simulink model "PIDcontroller"  (Simulink 6.5)
settings: Solver=FixedStepDiscrete  StartTime=0.0  StopTime=10.0  FixedStep=0.1  RelTol=1e-3
settings Model: Creator=AugustineBui  LastModifiedBy=AugustineBui
settings OptimizationCC: InitFltsAndDblsToZero=off
settings DebuggingCC: SignalResolutionControl=UseLocalSettings  StrictBusMsg=ErrorLevel1
settings HardwareCC: TargetHWDeviceType=32-bit Generic
settings GRTTargetCC: ExtModeInterfaceLevel=Level1

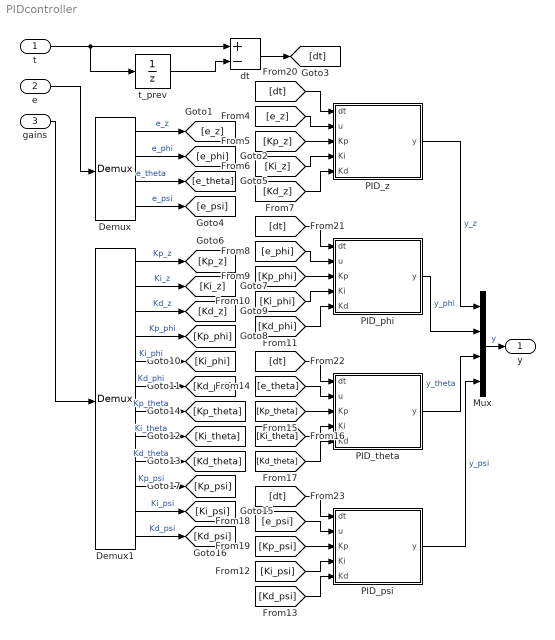
== system PIDcontroller ==
  t : Inport  PortDimensions=1  DataType=double
  e : Inport  Port=2  PortDimensions=4  DataType=double
  gains : Inport  Port=3  PortDimensions=12  DataType=double
  Demux : Demux
  Demux1 : Demux  Outputs=12
  Mux : Mux
  PID_phi : Subsystem
  PID_psi : Subsystem
  PID_theta : Subsystem
  PID_z : Subsystem
  dt : Sum  Inputs=+-
  t_prev : UnitDelay  X0=-0.5  SampleTime=-1
  y : Outport
  wires:
  [Kd_psi] -> PID_psi/5(Kd)
  [Ki_psi] -> PID_psi/4(Ki)
  [dt] -> PID_psi/1(dt)
  [e_psi] -> PID_psi/2(u)
  [Kp_psi] -> PID_psi/3(Kp)
  PID_psi/1(y) -> Mux/4  "y_psi"
  PID_theta/1(y) -> Mux/3  "y_theta"
  [Kd_theta] -> PID_theta/5(Kd)
  [Ki_theta] -> PID_theta/4(Ki)
  [dt] -> PID_theta/1(dt)
  [e_theta] -> PID_theta/2(u)
  [Kp_theta] -> PID_theta/3(Kp)
  PID_phi/1(y) -> Mux/2  "y_phi"
  [Kp_phi] -> PID_phi/3(Kp)
  [dt] -> PID_phi/1(dt)
  [dt] -> PID_z/1(dt)
  dt/1 -> [dt]
  [e_phi] -> PID_phi/2(u)
  t/1 -> t_prev/1, dt/1
  t_prev/1 -> dt/2
  e/1 -> Demux/1
  gains/1 -> Demux1/1
  Demux/1 -> [e_z]  "e_z"
  Demux/2 -> [e_phi]  "e_phi"
  Demux/3 -> [e_theta]  "e_theta"
  Demux/4 -> [e_psi]  "e_psi"
  Demux1/1 -> [Kp_z]  "Kp_z"
  Demux1/2 -> [Ki_z]  "Ki_z"
  Demux1/3 -> [Kd_z]  "Kd_z"
  Demux1/4 -> [Kp_phi]  "Kp_phi"
  Demux1/5 -> [Ki_phi]  "Ki_phi"
  Demux1/6 -> [Kd_phi]  "Kd_phi"
  Demux1/7 -> [Kp_theta]  "Kp_theta"
  Demux1/8 -> [Ki_theta]  "Ki_theta"
  Demux1/9 -> [Kd_theta]  "Kd_theta"
  Demux1/10 -> [Kp_psi]  "Kp_psi"
  Demux1/11 -> [Ki_psi]  "Ki_psi"
  Demux1/12 -> [Kd_psi]  "Kd_psi"
  [e_z] -> PID_z/2(u)
  [Kp_z] -> PID_z/3(Kp)
  [Ki_z] -> PID_z/4(Ki)
  [Kd_z] -> PID_z/5(Kd)
  PID_z/1(y) -> Mux/1  "y_z"
  [Ki_phi] -> PID_phi/4(Ki)
  [Kd_phi] -> PID_phi/5(Kd)
  Mux/1 -> y/1  "y"

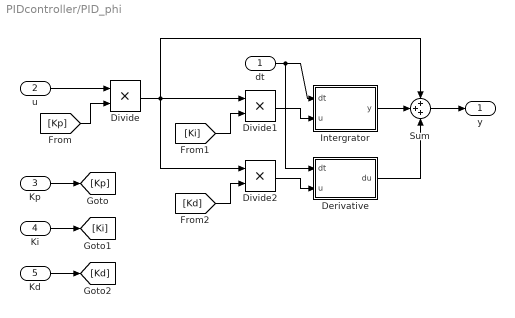
== system PIDcontroller/PID_phi ==
  dt : Inport
  u : Inport  Port=2
  Kp : Inport  Port=3
  Ki : Inport  Port=4
  Kd : Inport  Port=5
  Derivative : Subsystem
  Divide : Product  Inputs=**
  Divide1 : Product  Inputs=**
  Divide2 : Product  Inputs=**
  Intergrator : Subsystem
  Sum : Sum  Inputs=+++
  y : Outport
  wires:
  Kp/1 -> [Kp]
  Ki/1 -> [Ki]
  Kd/1 -> [Kd]
  [Kp] -> Divide/2
  u/1 -> Divide/1
  Divide/1 -> Divide1/1, Divide2/1, Sum/1
  [Ki] -> Divide1/2
  [Kd] -> Divide2/2
  Divide2/1 -> Derivative/2(u)
  Divide1/1 -> Intergrator/2(u)
  Intergrator/1(y) -> Sum/2
  Derivative/1(du) -> Sum/3
  Sum/1 -> y/1
  dt/1 -> Derivative/1(dt), Intergrator/1(dt)

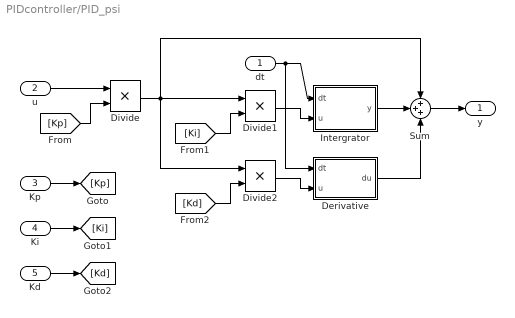
== system PIDcontroller/PID_psi ==
  dt : Inport
  u : Inport  Port=2
  Kp : Inport  Port=3
  Ki : Inport  Port=4
  Kd : Inport  Port=5
  Derivative : Subsystem
  Divide : Product  Inputs=**
  Divide1 : Product  Inputs=**
  Divide2 : Product  Inputs=**
  Intergrator : Subsystem
  Sum : Sum  Inputs=+++
  y : Outport
  wires:
  Kp/1 -> [Kp]
  Ki/1 -> [Ki]
  Kd/1 -> [Kd]
  [Kp] -> Divide/2
  u/1 -> Divide/1
  Divide/1 -> Divide1/1, Divide2/1, Sum/1
  [Ki] -> Divide1/2
  [Kd] -> Divide2/2
  Divide2/1 -> Derivative/2(u)
  Divide1/1 -> Intergrator/2(u)
  Intergrator/1(y) -> Sum/2
  Derivative/1(du) -> Sum/3
  Sum/1 -> y/1
  dt/1 -> Derivative/1(dt), Intergrator/1(dt)

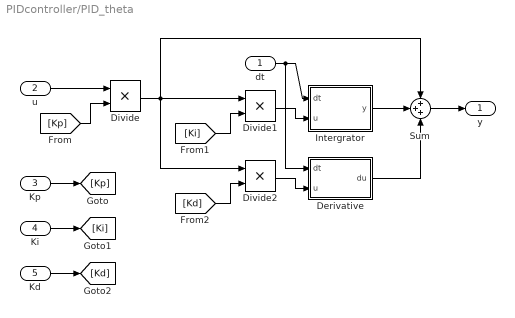
== system PIDcontroller/PID_theta ==
  dt : Inport
  u : Inport  Port=2
  Kp : Inport  Port=3
  Ki : Inport  Port=4
  Kd : Inport  Port=5
  Derivative : Subsystem
  Divide : Product  Inputs=**
  Divide1 : Product  Inputs=**
  Divide2 : Product  Inputs=**
  Intergrator : Subsystem
  Sum : Sum  Inputs=+++
  y : Outport
  wires:
  Kp/1 -> [Kp]
  Ki/1 -> [Ki]
  Kd/1 -> [Kd]
  [Kp] -> Divide/2
  u/1 -> Divide/1
  Divide/1 -> Divide1/1, Divide2/1, Sum/1
  [Ki] -> Divide1/2
  [Kd] -> Divide2/2
  Divide2/1 -> Derivative/2(u)
  Divide1/1 -> Intergrator/2(u)
  Intergrator/1(y) -> Sum/2
  Derivative/1(du) -> Sum/3
  Sum/1 -> y/1
  dt/1 -> Derivative/1(dt), Intergrator/1(dt)

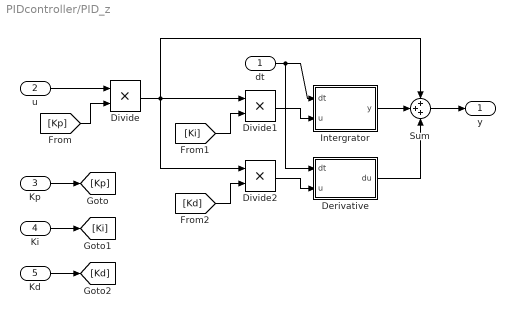
== system PIDcontroller/PID_z ==
  dt : Inport
  u : Inport  Port=2
  Kp : Inport  Port=3
  Ki : Inport  Port=4
  Kd : Inport  Port=5
  Derivative : Subsystem
  Divide : Product  Inputs=**
  Divide1 : Product  Inputs=**
  Divide2 : Product  Inputs=**
  Intergrator : Subsystem
  Sum : Sum  Inputs=+++
  y : Outport
  wires:
  Kp/1 -> [Kp]
  Ki/1 -> [Ki]
  Kd/1 -> [Kd]
  [Kp] -> Divide/2
  u/1 -> Divide/1
  Divide/1 -> Divide1/1, Divide2/1, Sum/1
  [Ki] -> Divide1/2
  [Kd] -> Divide2/2
  Divide2/1 -> Derivative/2(u)
  Divide1/1 -> Intergrator/2(u)
  Intergrator/1(y) -> Sum/2
  Derivative/1(du) -> Sum/3
  Sum/1 -> y/1
  dt/1 -> Intergrator/1(dt), Derivative/1(dt)

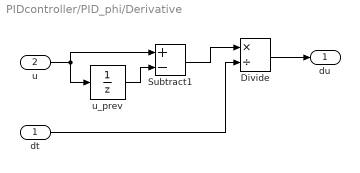
== system PIDcontroller/PID_phi/Derivative ==
  dt : Inport
  u : Inport  Port=2  PortDimensions=1  DataType=double
  Divide : Product  Inputs=*/
  Subtract1 : Sum  Inputs=+-
  u_prev : UnitDelay  SampleTime=-1
  du : Outport
  wires:
  u/1 -> u_prev/1, Subtract1/1
  u_prev/1 -> Subtract1/2
  Subtract1/1 -> Divide/1
  Divide/1 -> du/1
  dt/1 -> Divide/2

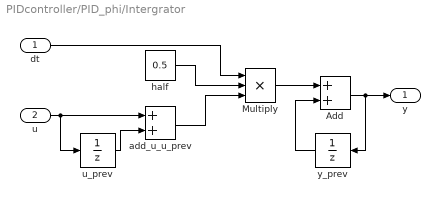
== system PIDcontroller/PID_phi/Intergrator ==
  dt : Inport  PortDimensions=1  DataType=double
  u : Inport  Port=2  PortDimensions=1  DataType=double
  Add : Sum
  Multiply : Product  Inputs=***
  add_u_u_prev : Sum
  half : Constant  Value=0.5
  u_prev : UnitDelay  SampleTime=-1
  y_prev : UnitDelay  Orientation=left  SampleTime=-1
  y : Outport
  wires:
  u/1 -> u_prev/1, add_u_u_prev/1
  Multiply/1 -> Add/1
  Add/1 -> y/1, y_prev/1
  y_prev/1 -> Add/2
  u_prev/1 -> add_u_u_prev/2
  add_u_u_prev/1 -> Multiply/3
  half/1 -> Multiply/2
  dt/1 -> Multiply/1

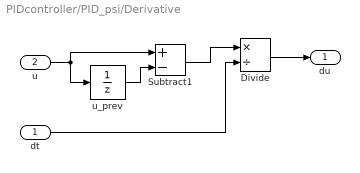
== system PIDcontroller/PID_psi/Derivative ==
  dt : Inport
  u : Inport  Port=2  PortDimensions=1  DataType=double
  Divide : Product  Inputs=*/
  Subtract1 : Sum  Inputs=+-
  u_prev : UnitDelay  SampleTime=-1
  du : Outport
  wires:
  u/1 -> u_prev/1, Subtract1/1
  u_prev/1 -> Subtract1/2
  Subtract1/1 -> Divide/1
  Divide/1 -> du/1
  dt/1 -> Divide/2

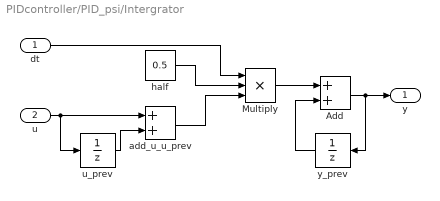
== system PIDcontroller/PID_psi/Intergrator ==
  dt : Inport  PortDimensions=1  DataType=double
  u : Inport  Port=2  PortDimensions=1  DataType=double
  Add : Sum
  Multiply : Product  Inputs=***
  add_u_u_prev : Sum
  half : Constant  Value=0.5
  u_prev : UnitDelay  SampleTime=-1
  y_prev : UnitDelay  Orientation=left  SampleTime=-1
  y : Outport
  wires:
  u/1 -> u_prev/1, add_u_u_prev/1
  Multiply/1 -> Add/1
  Add/1 -> y/1, y_prev/1
  y_prev/1 -> Add/2
  u_prev/1 -> add_u_u_prev/2
  add_u_u_prev/1 -> Multiply/3
  half/1 -> Multiply/2
  dt/1 -> Multiply/1

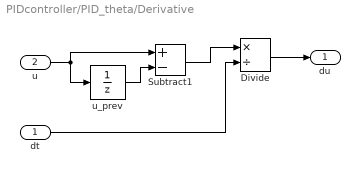
== system PIDcontroller/PID_theta/Derivative ==
  dt : Inport
  u : Inport  Port=2  PortDimensions=1  DataType=double
  Divide : Product  Inputs=*/
  Subtract1 : Sum  Inputs=+-
  u_prev : UnitDelay  SampleTime=-1
  du : Outport
  wires:
  u/1 -> u_prev/1, Subtract1/1
  u_prev/1 -> Subtract1/2
  Subtract1/1 -> Divide/1
  Divide/1 -> du/1
  dt/1 -> Divide/2

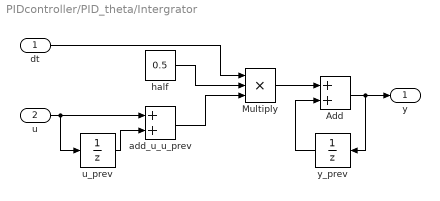
== system PIDcontroller/PID_theta/Intergrator ==
  dt : Inport  PortDimensions=1  DataType=double
  u : Inport  Port=2  PortDimensions=1  DataType=double
  Add : Sum
  Multiply : Product  Inputs=***
  add_u_u_prev : Sum
  half : Constant  Value=0.5
  u_prev : UnitDelay  SampleTime=-1
  y_prev : UnitDelay  Orientation=left  SampleTime=-1
  y : Outport
  wires:
  u/1 -> u_prev/1, add_u_u_prev/1
  Multiply/1 -> Add/1
  Add/1 -> y/1, y_prev/1
  y_prev/1 -> Add/2
  u_prev/1 -> add_u_u_prev/2
  add_u_u_prev/1 -> Multiply/3
  half/1 -> Multiply/2
  dt/1 -> Multiply/1

== system PIDcontroller/PID_z/Derivative ==
  dt : Inport
  u : Inport  Port=2  PortDimensions=1  DataType=double
  Divide : Product  Inputs=*/
  Subtract1 : Sum  Inputs=+-
  u_prev : UnitDelay  SampleTime=-1
  du : Outport
  wires:
  u/1 -> u_prev/1, Subtract1/1
  u_prev/1 -> Subtract1/2
  Subtract1/1 -> Divide/1
  Divide/1 -> du/1
  dt/1 -> Divide/2

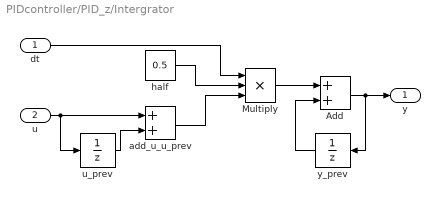
== system PIDcontroller/PID_z/Intergrator ==
  dt : Inport  PortDimensions=1  DataType=double
  u : Inport  Port=2  PortDimensions=1  DataType=double
  Add : Sum
  Multiply : Product  Inputs=***
  add_u_u_prev : Sum
  half : Constant  Value=0.5
  u_prev : UnitDelay  SampleTime=-1
  y_prev : UnitDelay  Orientation=left  SampleTime=-1
  y : Outport
  wires:
  u/1 -> u_prev/1, add_u_u_prev/1
  Multiply/1 -> Add/1
  Add/1 -> y/1, y_prev/1
  y_prev/1 -> Add/2
  u_prev/1 -> add_u_u_prev/2
  add_u_u_prev/1 -> Multiply/3
  half/1 -> Multiply/2
  dt/1 -> Multiply/1
